simulink model "abs_main"  (R2024b)
settings: Solver=ode15s  StartTime=0.0  StopTime=10  RelTol=1e-3
settings Model: Creator=rocke  LastModifiedBy=rocke

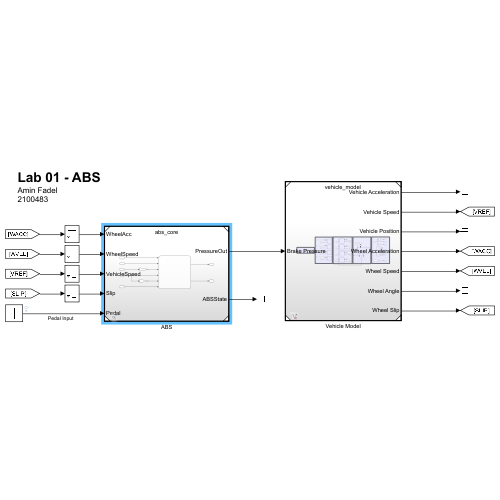
[thumbnail: Simulink's stored preview of the top-level diagram]
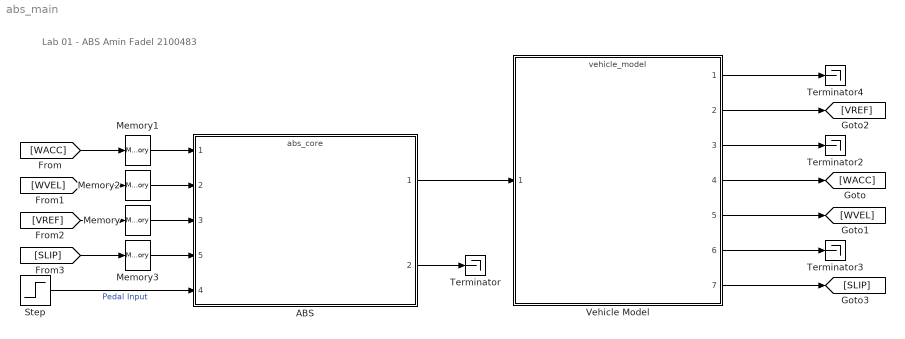
== system abs_main ==
  note: Lab 01 - ABS
      | Amin Fadel
      | 2100483
  ABS : ModelReference  ModelNameDialog=abs_core  SimulationMode=Normal  ModelReferenceVersion=1.28
      settings: PortSchema="{\"entries\":[{\"content\":{\"sides\":[{\"content\":{\"connectorIds\":[\"In1\",\"In2\",\"In3\",\"In5\",\"In4\"]},\"type\":\"ConnectorPlacement.EquallySpacedRectSide\",\"uuid\":\"0ef8b3d8-a5af-469c-bd39-588f71cde844\"},{\"content\":{\"connectorIds\":[\"Out1\",\"Out2\"],\"side\":\"RIGHT\"},\"type\":\"ConnectorPlacement.EquallySpacedRectSide\",\"uuid\":\"5bda9995-afda-4d01-80e2-9489bdcbf6b0\"},{\"content\":{\"side\":\"TOP\"},\"type\":\"ConnectorPlacement.EquallySpacedRectSide\",\"uuid\":\"848c1bd4-65ec-438a-8a48-1fb20937bff8\"}]},\"type\":\"ConnectorPlacement.EquallySpacedConnector\",\"uuid\":\"20e0b17e-623b-4232-9650-d93f1a785f62\"}],\"packageUris\":[\"http://schema.mathworks.com/mf0/Connector/R2020b\"],\"version\":\"1.0\"}"
  Memory{,1..3} (4 alike) : Memory
  Step : Step  SampleTime=0
  Terminator{,2..4} (4 alike) : Terminator
  Vehicle Model : ModelReference  ModelNameDialog=vehicle_model  SimulationMode=Normal  ModelReferenceVersion=1.10
  wires:
  ABS/1 -> Vehicle Model/1
  Vehicle Model/4 -> [WACC]
  [WACC] -> Memory1/1
  Memory1/1 -> ABS/1
  Vehicle Model/5 -> [WVEL]
  Vehicle Model/2 -> [VREF]
  [WVEL] -> Memory2/1
  Memory2/1 -> ABS/2
  [VREF] -> Memory/1
  Memory/1 -> ABS/3
  Step/1 -> ABS/4  "Pedal Input"
  ABS/2 -> Terminator/1
  Vehicle Model/7 -> [SLIP]
  Vehicle Model/6 -> Terminator3/1
  Vehicle Model/3 -> Terminator2/1
  Vehicle Model/1 -> Terminator4/1
  [SLIP] -> Memory3/1
  Memory3/1 -> ABS/5
